simulink model "TrafficLightTemplate"  (R2017b)
settings: Solver=VariableStepAuto  StartTime=0.0  StopTime=inf  RelTol=1e-3
settings Model: Creator=davit  LastModifiedBy=Nitin

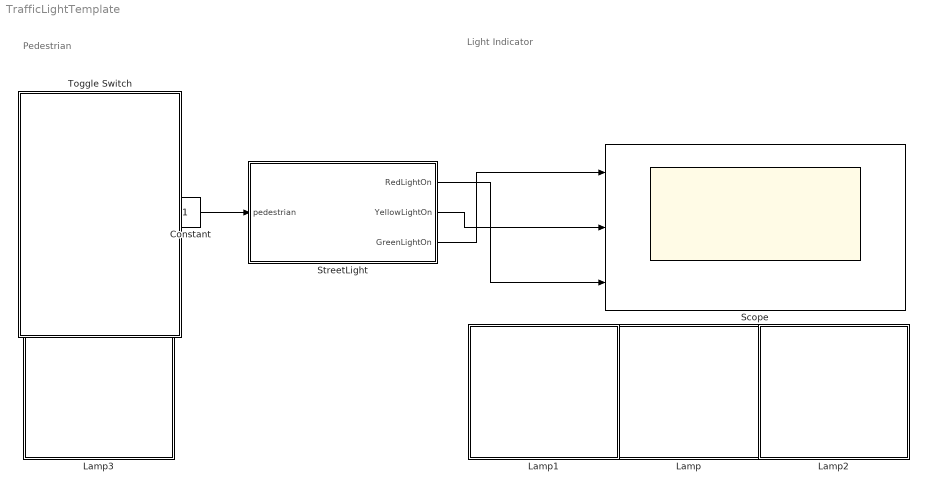
== system TrafficLightTemplate ==
  note: Pedestrian
  note: Light Indicator
  Constant : Constant  OutDataTypeStr=boolean
  Lamp : Subsystem  DialogController=hmiCreateDDGDialog  IsWebBlock=on  mask(MWDashboardBlock){webBlockId=09f4af96-59e9-4a04-926b-3f38731730af, webBlockType=lamp, ShowInLibBrowser=on, ShowInitialText=on, HMISrcModelName=zantouts_TrafficLightTemplate}
      mask prompts: webBlockType "WebBlock Type"; HMISrcModelName "Source Model"
      mask help: SimulinkHMI:dialogs:LampDialogDesc
      mask Help: helpview([docroot '/mapfiles/simulink.map'], 'hmi_lamp')
      mask Display:
      | if strcmp(get_param(bdroot(gcb),'BlockDiagramType'), 'library')
      |     image([(matlabroot) '/toolbox/simulink/hmi/icons/Lamp.png']);
      | end
  Lamp1 : Subsystem  DialogController=hmiCreateDDGDialog  IsWebBlock=on  mask(MWDashboardBlock){webBlockId=13e3d59b-7669-4874-9118-3aee051ed5bc, webBlockType=lamp, ShowInLibBrowser=on, ShowInitialText=on, HMISrcModelName=zantouts_TrafficLightTemplate}
      mask prompts: webBlockType "WebBlock Type"; HMISrcModelName "Source Model"
      mask help: SimulinkHMI:dialogs:LampDialogDesc
      mask Help: helpview([docroot '/mapfiles/simulink.map'], 'hmi_lamp')
      mask Display:
      | if strcmp(get_param(bdroot(gcb),'BlockDiagramType'), 'library')
      |     image([(matlabroot) '/toolbox/simulink/hmi/icons/Lamp.png']);
      | end
  Lamp2 : Subsystem  DialogController=hmiCreateDDGDialog  IsWebBlock=on  mask(MWDashboardBlock){webBlockId=45cf720e-54e6-4924-aaf3-f56a1f358a4e, webBlockType=lamp, ShowInLibBrowser=on, ShowInitialText=on, HMISrcModelName=zantouts_TrafficLightTemplate}
      mask prompts: webBlockType "WebBlock Type"; HMISrcModelName "Source Model"
      mask help: SimulinkHMI:dialogs:LampDialogDesc
      mask Help: helpview([docroot '/mapfiles/simulink.map'], 'hmi_lamp')
      mask Display:
      | if strcmp(get_param(bdroot(gcb),'BlockDiagramType'), 'library')
      |     image([(matlabroot) '/toolbox/simulink/hmi/icons/Lamp.png']);
      | end
  Lamp3 : Subsystem  DialogController=hmiCreateDDGDialog  IsWebBlock=on  mask(MWDashboardBlock){webBlockId=06c2ae42-b6f6-477e-b988-39d56db1683e, webBlockType=lamp, ShowInLibBrowser=on, ShowInitialText=on, HMISrcModelName=zantouts_TrafficLightTemplate}
      mask prompts: webBlockType "WebBlock Type"; HMISrcModelName "Source Model"
      mask help: SimulinkHMI:dialogs:LampDialogDesc
      mask Help: helpview([docroot '/mapfiles/simulink.map'], 'hmi_lamp')
      mask Display:
      | if strcmp(get_param(bdroot(gcb),'BlockDiagramType'), 'library')
      |     image([(matlabroot) '/toolbox/simulink/hmi/icons/Lamp.png']);
      | end
  Scope : Scope  NumInputPorts=3
  StreetLight : Stateflow chart  TreatAsAtomicUnit=on
  Toggle Switch : Subsystem  DialogController=hmiCreateDDGDialog  IsWebBlock=on  mask(MWDashboardBlock){webBlockId=1ab5a5c0-b2ce-4713-9aaf-e6477c433adb, webBlockType=toggleswitch, ShowInLibBrowser=on, ShowInitialText=on, HMISrcModelName=zantouts_TrafficLightTemplate}
      mask prompts: webBlockId "WebBlock Id"; webBlockType "WebBlock Type"; HMISrcModelName "Source Model"
      mask help: SimulinkHMI:dialogs:SwitchDialogDesc
      mask Help: helpview([docroot '/mapfiles/simulink.map'], 'hmi_toggle_switch')
      mask Display:
      | if strcmp(get_param(bdroot(gcb),'BlockDiagramType'), 'library')
      |     image([(matlabroot) '/toolbox/simulink/hmi/icons/ToggleSwitch.png']);
      | end
  wires:
  Constant/1 -> StreetLight/1(pedestrian)
  StreetLight/1(RedLightOn) -> Scope/3
  StreetLight/3(GreenLightOn) -> Scope/1
  StreetLight/2(YellowLightOn) -> Scope/2

== system TrafficLightTemplate/Lamp ==

== system TrafficLightTemplate/Lamp1 ==

== system TrafficLightTemplate/Lamp2 ==

== system TrafficLightTemplate/Lamp3 ==

== system TrafficLightTemplate/Toggle Switch ==

== stateflow chart TrafficLightTemplate/StreetLight ==
  settings: executeAtInitialization=1
  state Red
    entry:RedLightOn=1;
    exit:RedLightOn=0;
  state Green
    entry:GreenLightOn=1;
    exit:GreenLightOn=0;
  state Yellow
    entry: YellowLightOn = 1;
    exit: YellowLightOn = 0;
  (default) -> Red : {counter=0;}
  Red -> Red [order 2] : [counter<10]{counter=counter+1;pause(1);}
  Green -> Green [order 3] : [(pedestrian==0 && counter<10) || (pedestrian ==1 && counter <20)]{pause(1);counter=counter+1}
  Red -> Green [order 1] : [counter==10]{counter=0;}
  Green -> Yellow [order 1] : [pedestrian == 0 && counter==20]{counter=0}
  Green -> Yellow [order 2] : [pedestrian == 1 & counter==20]{counter=0;}
  Yellow -> Red [order 1] : [counter==3]{counter=0}
  Yellow -> Yellow [order 2] : [counter<3]{pause(1);counter=counter+1;}
  data: RedLightOn output; YellowLightOn output; GreenLightOn output; pedestrian input boolean =false; counter local
